simulink model "superTwisting"  (R2023a)
settings: Solver=FixedStepAuto  StartTime=0.0  StopTime=10  FixedStep=0.0001  RelTol=1e-3
settings Model: Creator=headl  LastModifiedBy=headl

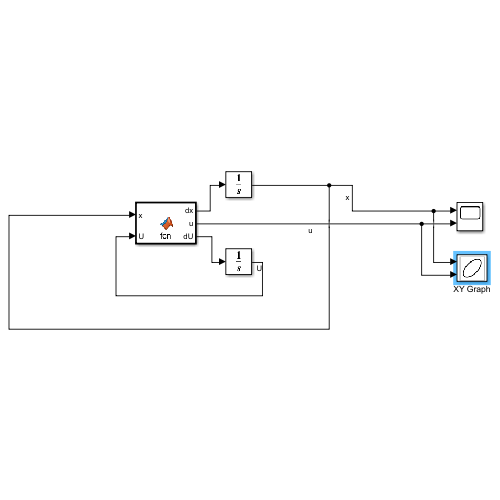
[thumbnail: Simulink's stored preview of the top-level diagram]
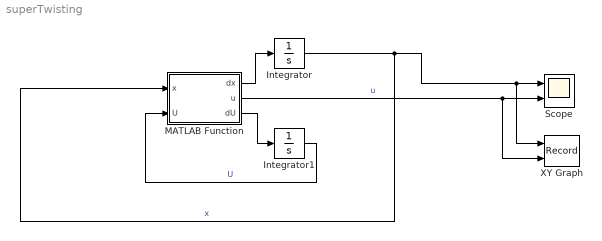
== system superTwisting ==
  Integrator : Integrator  InitialCondition=pi/3
  Integrator1 : Integrator
  MATLAB Function : MATLAB Function  TreatAsAtomicUnit=on
  Scope : Scope  NumInputPorts=2
  XY Graph : Record  FileSettingsInternal="{\"entries\":[{\"content\":{\"excelSettings\":{\"content\":{},\"type\":\"Streamout.ExcelSettings\"}},\"type\":\"Streamout.FileSettingStorage\",\"uuid\":\"\"}],\"packageUris\":[\"http:\\/\\/schema.mathworks.com\\/mf0\\/streamout_blocks\\/R2020a\"],\"version\":\"1.0\"}"  Layout=[1 1]  SignalsInternal="{\"entries\":[{\"content\":{\"signals\":[{\"content\":{\"blockPath\":[],\"dimensions\":[1],\"domain\":\"\",\"lineColor\":\"#a2142f\",\"plots\":[1],\"port\":1,\"sid\":[\"\"],\"signalID\":607,\"signalName\":\"x\"},\"type\":\"RecordBlkView.Signal\",\"uuid\":\"\"},{\"content\":{\"blockPath\":[],\"dimensions\":[1],\"domain\":\"\",\"lineColor\":\"#139fff\",\"plots\":[1],\"port\":2,\"sid\":[\"\"],\"signalID\":611,\"signalName\":\"u\"},\"type\":\"RecordBlkView.Signal\",\"uuid\":\"\"}]},\"type\":\"RecordBlkView.InputSignals\",\"uuid\":\"\"}],\"packageUris\":[\"http:\\/\\/schema.mathworks.com\\/mf0\\/streamout_blocks\\/R2020a\"],\"version\":\"1.0\"}"  VisualizationBindings="{\"xyplotplugin\":{\"info\":[{\"series\":[{\"bindingParametersList\":[{\"parameter\":\"X-Axis\",\"signalID\":607,\"signalName\":\"x\"},{\"parameter\":\"Y-Axis\",\"signalID\":611,\"signalName\":\"u\"}],\"seriesID\":22895}],\"subplotID\":1}]}}"  CompatibilityTag=XY
  wires:
  MATLAB Function/1(dx) -> Integrator/1
  Integrator/1 -> MATLAB Function/1(x), XY Graph/1, Scope/1  "x"
  MATLAB Function/3(dU) -> Integrator1/1
  Integrator1/1 -> MATLAB Function/2(U)  "U"
  MATLAB Function/2(u) -> XY Graph/2, Scope/2  "u"

== matlab function superTwisting/MATLAB Function ==
  data: x input; dx output; u output; U input; dU output
function [dx,u, dU] = fcn(x,U)

q = pi/6;

if abs(U) > 1
    dU = -U;
else
    dU = -2*sign(x);
end

%u = -2*sign(x);
u = U;
%u = 0;

dx = -sin(x+q) + u;
